simulink model "non_linear_model_block"  (R2024b)
settings: Solver=VariableStepAuto  StartTime=0.0  StopTime=50  MaxStep=0.01  RelTol=1e-3
values from neighbouring files (symbols this model uses):
  a1 = sqrt(2*g)    [param_identification.m]    (also in simulation_parameters.m = A_out/A_t*sqrt(2*g/(1+zeta)))
  a2 = mean(a2)    [param_identification.m]    (also in simulation_parameters.m = 0.0216)
  A_t = 50e2    (= 5000)    [simulation_parameters.m]    (also in simulation_parameters_simple.m = 5e-05)
  K_pump = 1000    [simulation_parameters.m]    (also in simulation_parameters_simple.m = 0.0166666667)
  rho = 997    [simulation_parameters.m]    (also in simulation_parameters_simple.m)
  u0 = 1/4    (= 0.25)    [simulation_parameters.m]    (also in simulation_parameters_simple.m)
libraries: slpidlib x1
settings Model: Creator=andit  LastModifiedBy=andit

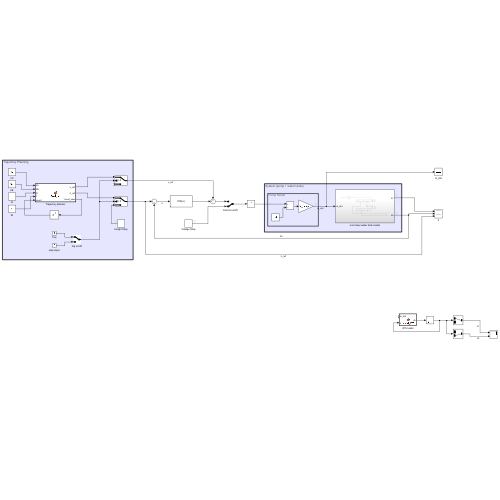
[thumbnail: Simulink's stored preview of the top-level diagram]
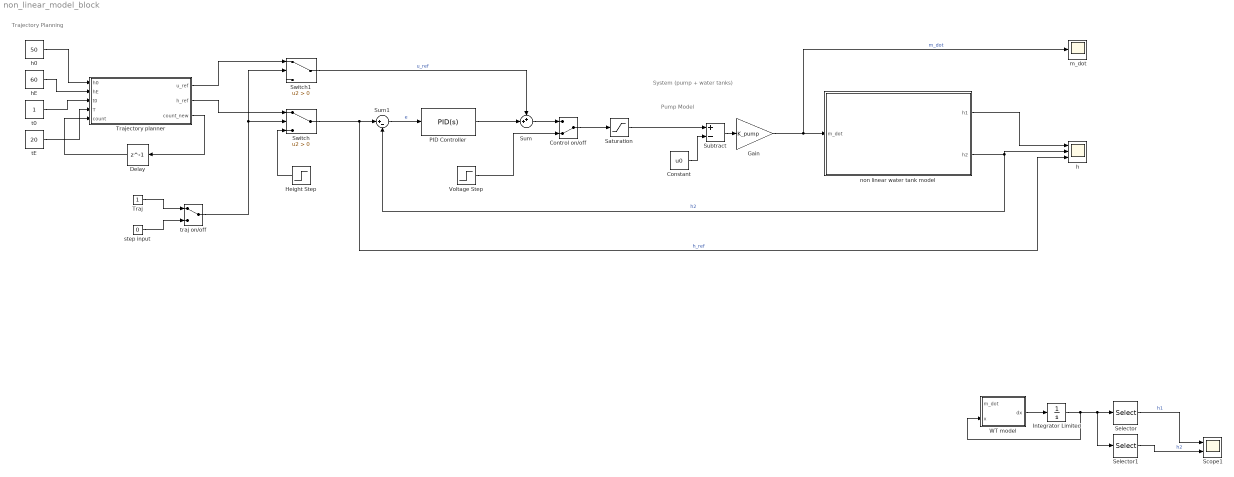
== system non_linear_model_block ==
  note: Trajectory Planning
  note: System (pump + water tanks)
  note: Pump Model
  Constant : Constant  Value=u0
  Control on/off : ManualSwitch  CurrentSetting=0
  Delay : Delay  DelayLength=1
  Gain : Gain  Gain=K_pump
  Height Step : Step  After=50  SampleTime=0
  Integrator Limited : Integrator  LimitOutput=on  UpperSaturationLimit=[300, 300]'  LowerSaturationLimit=0
  PID Controller : slpidlib/PID Controller  Controller=PID  Form=Parallel  TimeDomain=Continuous-time  UseExternalTs=off  SampleTime=-1  IntegratorMethod=Forward Euler  FilterMethod=Forward Euler  ControllerParametersSource=internal  P=1  I=1  UseKiTs=off  D=0  UseExternalDerivativeSource=off  N=100  UseFilter=on  TunerSelectOption=Transfer Function Based (PID Tuner App)  InitialConditionSource=internal  InitialConditionForIntegrator=0  InitialConditionForFilter=0  DifferentiatorICPrevScaledInput=0  ExternalReset=none  TrackingMode=off  Kt=1  LimitOutput=off  SatLimitsSource=internal  UpperSaturationLimit=inf  LowerSaturationLimit=-inf  LinearizeAsGain=on  AntiWindupMode=none  Kb=1  LimitIntegrator=off  UpperIntegratorSaturationLimit=inf  LowerIntegratorSaturationLimit=-inf  POutMin=[]  POutMax=[]  IOutMin=[]  IOutMax=[]  DOutMin=[]  DOutMax=[]  NOutMin=[]  NOutMax=[]  SumOutMin=[]  SumOutMax=[]  SaturationOutMin=[]  SaturationOutMax=[]  PParamMin=[]  PParamMax=[]  IParamMin=[]  IParamMax=[]  DParamMin=[]  DParamMax=[]  NParamMin=[]  NParamMax=[]  KbParamMin=[]  KbParamMax=[]  KtParamMin=[]  KtParamMax=[]  KbOutMin=[]  KbOutMax=[]  KtOutMin=[]  KtOutMax=[]  IntegratorOutMin=[]  IntegratorOutMax=[]  FilterOutMin=[]  FilterOutMax=[]  SumI1OutMin=[]  SumI1OutMax=[]  SumI2OutMin=[]  SumI2OutMax=[]  SumI3OutMin=[]  SumI3OutMax=[]  SumI4OutMin=[]  SumI4OutMax=[]  SumDOutMin=[]  SumDOutMax=[]  DifferentiatorOutMin=[]  DifferentiatorOutMax=[]  FilterDiffOutCoefMin=[]  FilterDiffOutCoefMax=[]  ReciprocalOutMin=[]  ReciprocalOutMax=[]  SumDenOutMin=[]  SumDenOutMax=[]  SumNumOutMin=[]  SumNumOutMax=[]  DivideOutMin=[]  DivideOutMax=[]  UdiffTsProdOutMin=[]  UdiffTsProdOutMax=[]  NTsProdOutMin=[]  NTsProdOutMax=[]  UintegralTsProdOutMin=[]  UintegralTsProdOutMax=[]  UngainTsProdOutMin=[]  UngainTsProdOutMax=[]  ClampingZeroOutDataTypeStr=Inherit: Inherit via back propagation  ClampingZeroOutMin=[]  ClampingZeroOutMax=[]  FilterDenConstantOutDataTypeStr=Inherit: Inherit via back propagation  FilterDenConstantOutMin=[]  FilterDenConstantOutMax=[]  PCopyOutDataTypeStr=Inherit: Inherit via back propagation  PCopyOutMin=[]  PCopyOutMax=[]  NCopyOutDataTypeStr=Inherit: Inherit via back propagation  NCopyOutMin=[]  NCopyOutMax=[]  IntegratorContinuousStateAttributes=''  IntegratorStateMustResolveToSignalObject=off  IntegratorRTWStateStorageClass=Auto  FilterContinuousStateAttributes=''  FilterStateMustResolveToSignalObject=off  FilterRTWStateStorageClass=Auto  ParallelPVariant=InternalParameters  IdealPVariant=Disabled  IVariant=InternalParameters  DVariant=InternalParameters  IntegratorVariant=Continuous  SatVariant=Disabled  AWVariant=Passthrough  PCopyVariant=Disabled  TRVariant=Disabled  FdbkBlocksVariant=Forward  IdealPFdbkVariant=Disabled  SatFdbkVariant=Disabled  DerivativeFilterVariant=ContFilter  NVariant=InternalParameters  NCopyVariant=Disabled  FilterICVariant=InternalICsFilter  IntegratorICVariant=InternalICs  ExternalResetVariant=Disabled  TRSumVariant=Passthrough  SumFdbkVariant=Disabled  SumVariant=Sum_PID  TsampFilterVariant=InternalTs  TsampNgainVariant=Passthrough  TsampIntegralVariant=Disabled_SignalSpec  ExternalSaturationOutDataTypeStr=Inherit: Same as second input  DerivativeSourceVariant=ErrorSignal  PreIntVariant=InternalPreInt
  Saturation : Saturate  UpperLimit=5  LowerLimit=0
  Scope1 : Scope  NumInputPorts=2
  Selector : Selector  InputPortWidth=2  IndexOptions=Index vector (dialog)  Indices=[1]  OutputSizes=1
  Selector1 : Selector  InputPortWidth=2  IndexOptions=Index vector (dialog)  Indices=[2]  OutputSizes=1
  Subtract : Sum  Inputs=+-
  Sum : Sum  Inputs=++|
  Sum1 : Sum  Inputs=|+-
  Switch : Switch  Criteria=u2 > Threshold  SaturateOnIntegerOverflow=off  InputSameDT=off
  Switch1 : Switch  Criteria=u2 > Threshold  SaturateOnIntegerOverflow=off  InputSameDT=off
  Traj : Constant
  Trajectory planner : MATLAB Function  TreatAsAtomicUnit=on
  Voltage Step : Step  After=4  SampleTime=0
  WT model : MATLAB Function  TreatAsAtomicUnit=on
  h : Scope  NumInputPorts=3
  h0 : Constant  Value=50
  hE : Constant  Value=60
  m_dot : Scope
  non linear water tank model : Subsystem
  step input : Constant  Value=0
  t0 : Constant
  tE : Constant  Value=20
  traj on/off : ManualSwitch
  wires:
  non linear water tank model/1(h1) -> h/1
  non linear water tank model/2(h2) -> h/2, Sum1/2  "h2"
  WT model/1(dx) -> Integrator Limited/1
  Integrator Limited/1 -> WT model/2(x), Selector1/1, Selector/1
  Selector/1 -> Scope1/1  "h1"
  Selector1/1 -> Scope1/2  "h2"
  Subtract/1 -> Gain/1
  Constant/1 -> Subtract/2
  Gain/1 -> m_dot/1, non linear water tank model/1(m_dot)  "m_dot"
  PID Controller/1 -> Sum/2
  Sum1/1 -> PID Controller/1  "e"
  Switch/1 -> h/3, Sum1/1  "h_ref"
  Trajectory planner/2(h_ref) -> Switch/1
  traj on/off/1 -> Switch/2, Switch1/2
  Trajectory planner/1(u_ref) -> Switch1/1
  Switch1/1 -> Sum/1  "u_ref"
  step input/1 -> traj on/off/2
  Traj/1 -> traj on/off/1
  Sum/1 -> Control on/off/1
  h0/1 -> Trajectory planner/1(h0)
  hE/1 -> Trajectory planner/2(hE)
  t0/1 -> Trajectory planner/3(t0)
  tE/1 -> Trajectory planner/4(T)
  Trajectory planner/3(count_new) -> Delay/1
  Delay/1 -> Trajectory planner/5(count)
  Control on/off/1 -> Saturation/1
  Saturation/1 -> Subtract/1
  Voltage Step/1 -> Control on/off/2
  Height Step/1 -> Switch/3

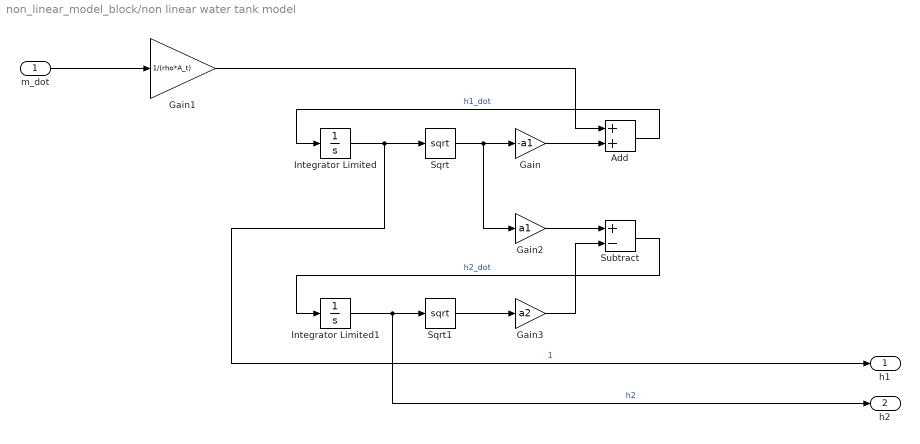
== system non_linear_model_block/non linear water tank model ==
  m_dot : Inport
  Add : Sum
  Gain : Gain  Gain=-a1
  Gain1 : Gain  Gain=1/(rho*A_t)
  Gain2 : Gain  Gain=a1
  Gain3 : Gain  Gain=a2
  Integrator Limited : Integrator  LimitOutput=on  UpperSaturationLimit=300  LowerSaturationLimit=0
  Integrator Limited1 : Integrator  LimitOutput=on  UpperSaturationLimit=300  LowerSaturationLimit=0
  Sqrt : Sqrt
  Sqrt1 : Sqrt
  Subtract : Sum  Inputs=+-
  h1 : Outport
  h2 : Outport  Port=2
  wires:
  Add/1 -> Integrator Limited/1  "h1_dot"
  Gain2/1 -> Subtract/1
  Integrator Limited/1 -> h1/1, Sqrt/1  "1"
  Integrator Limited1/1 -> h2/1, Sqrt1/1  "h2"
  Gain/1 -> Add/2
  Sqrt/1 -> Gain2/1, Gain/1
  Sqrt1/1 -> Gain3/1
  Gain3/1 -> Subtract/2
  Subtract/1 -> Integrator Limited1/1  "h2_dot"
  Gain1/1 -> Add/1
  m_dot/1 -> Gain1/1

== matlab function non_linear_model_block/Trajectory planner ==
  data: u_ref output; h_ref output; h0 input; hE input; t0 input; T input; count input; count_new output
function [u_ref, h_ref, count_new] = feed_fw(h0, hE, t0, T, count)

count_new = count+1;
dT = 0.1;         % passt dia NOOOOOOOOOOOOO?
t = count_new*dT-t0;

u_ref = 0;
h_ref = 0;


end

== matlab function non_linear_model_block/WT model ==
  data: m_dot input; dx output; x input
function dx  = model_WT(m_dot,x)

a1 = 0.0216;
a2 = 0.0216;
rho = 997;

h1_bar = 50;
h2_bar = 50;        
A_t = 50e2; % mm^2


h1 = x(1);
h2 = x(2);

dx = zeros(2,1);

dx(1) = -a1*sqrt(h1) + 1/(rho*A_t)*m_dot;
dx(2) = a1*sqrt(h1) - a2*sqrt(h2);

end
